simulink model "meter_TO_feet"  (R2021a)
settings: Solver=VariableStepAuto  StartTime=0.0  StopTime=10.0  RelTol=1e-3
settings Model: Creator=MAC  LastModifiedBy=MAC

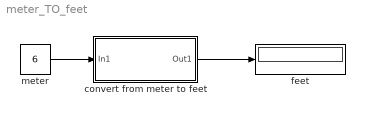
== system meter_TO_feet ==
  convert from meter to feet : Subsystem
  feet : Display
  meter : Constant  Value=6
  wires:
  meter/1 -> convert from meter to feet/1(In1)
  convert from meter to feet/1(Out1) -> feet/1

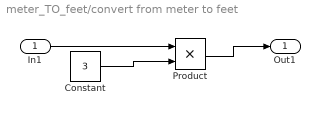
== system meter_TO_feet/convert from meter to feet ==
  In1 : Inport
  Constant : Constant  Value=3
  Product : Product
  Out1 : Outport
  wires:
  In1/1 -> Product/1
  Product/1 -> Out1/1
  Constant/1 -> Product/2
